simulink model "control_nonlinear"  (R2022b)
settings: Solver=VariableStepAuto  StartTime=0.0  StopTime=10.0  RelTol=1e-3
undefined symbols (not defined in the file or in its folder): magnitude
settings Model: Creator=integzz  LastModifiedBy=integzz

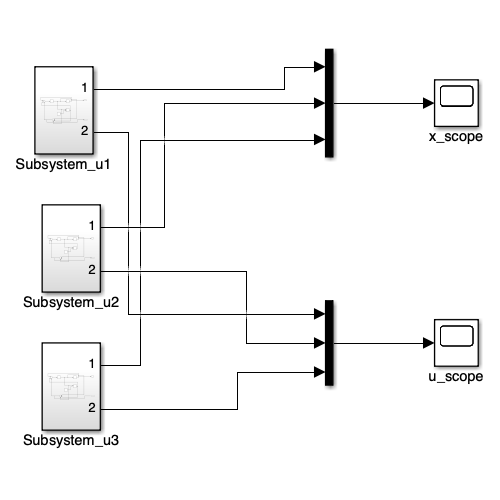
[thumbnail: Simulink's stored preview of the top-level diagram]
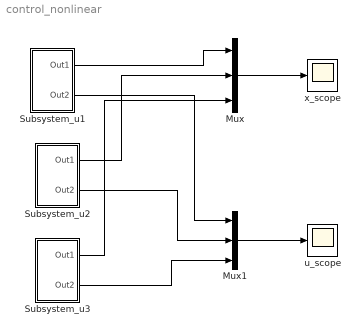
== system control_nonlinear ==
  Mux : Mux  Inputs=3
  Mux1 : Mux  Inputs=3
  Subsystem_u1 : Subsystem
  Subsystem_u2 : Subsystem
  Subsystem_u3 : Subsystem
  u_scope : Scope
  x_scope : Scope
  wires:
  Subsystem_u1/1(Out1) -> Mux/1
  Subsystem_u1/2(Out2) -> Mux1/1
  Mux/1 -> x_scope/1
  Mux1/1 -> u_scope/1
  Subsystem_u2/1(Out1) -> Mux/2
  Subsystem_u2/2(Out2) -> Mux1/2
  Subsystem_u3/1(Out1) -> Mux/3
  Subsystem_u3/2(Out2) -> Mux1/3

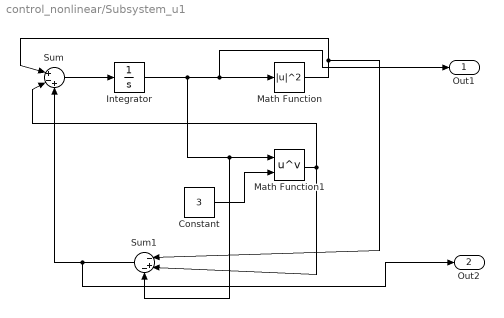
== system control_nonlinear/Subsystem_u1 ==
  Constant : Constant  Value=3
  Integrator : Integrator  InitialCondition=10
  Math Function : Math  Operator=magnitude^2
  Math Function1 : Math  Operator=pow
  Sum : Sum  Inputs=|+-+
  Sum1 : Sum  Inputs=|-+-
  Out1 : Outport
  Out2 : Outport  Port=2
  wires:
  Sum/1 -> Integrator/1
  Constant/1 -> Math Function1/2
  Math Function1/1 -> Sum1/2, Sum/2
  Sum1/1 -> Out2/1, Sum/3
  Math Function/1 -> Sum1/1, Sum/1
  Integrator/1 -> Math Function1/1, Sum1/3, Out1/1, Math Function/1

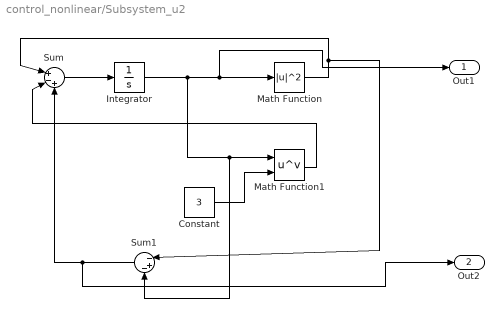
== system control_nonlinear/Subsystem_u2 ==
  Constant : Constant  Value=3
  Integrator : Integrator  InitialCondition=10
  Math Function : Math  Operator=magnitude^2
  Math Function1 : Math  Operator=pow
  Sum : Sum  Inputs=|+-+
  Sum1 : Sum  Inputs=|-+-
  Out1 : Outport
  Out2 : Outport  Port=2
  wires:
  Integrator/1 -> Math Function/1, Out1/1, Sum1/3, Math Function1/1
  Math Function/1 -> Sum/1, Sum1/1
  Sum1/1 -> Sum/3, Out2/1
  Math Function1/1 -> Sum/2
  Constant/1 -> Math Function1/2
  Sum/1 -> Integrator/1

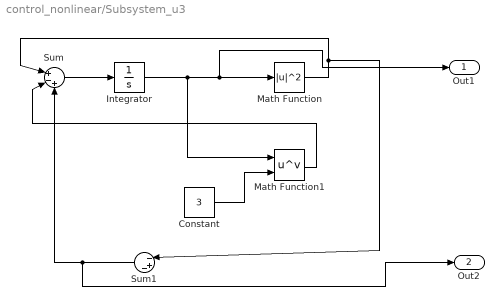
== system control_nonlinear/Subsystem_u3 ==
  Constant : Constant  Value=3
  Integrator : Integrator  InitialCondition=10
  Math Function : Math  Operator=magnitude^2
  Math Function1 : Math  Operator=pow
  Sum : Sum  Inputs=|+-+
  Sum1 : Sum  Inputs=|-+-
  Out1 : Outport
  Out2 : Outport  Port=2
  wires:
  Sum/1 -> Integrator/1
  Constant/1 -> Math Function1/2
  Math Function1/1 -> Sum/2
  Sum1/1 -> Out2/1, Sum/3
  Math Function/1 -> Sum1/1, Sum/1
  Integrator/1 -> Math Function1/1, Out1/1, Math Function/1
